simulink model "mw_autodma"  (R2020a)
settings: Solver=VariableStepAuto  StartTime=0.0  StopTime=(2*8192)/256e6  RelTol=1e-3
InitFcn:
  | fs = 256e6;
libraries: hdlsllib x5, simulink x4
settings Model: Creator=david  LastModifiedBy=david
settings OptimizationCC: BlockReduction=off  ConditionallyExecuteInputs=off  DefaultParameterBehavior=Inlined
settings DebuggingCC: AlgebraicLoopMsg=error
settings HardwareCC: ProdBitPerPointer=32  ProdBitPerSizeT=32  ProdBitPerPtrDiffT=32  ProdLargestAtomicFloat=None  ProdIntDivRoundTo=Undefined  ProdEndianess=Unspecified  ProdWordSize=32  ProdHWDeviceType=ASIC/FPGA->ASIC/FPGA  TargetBitPerPointer=64  TargetBitPerSizeT=64  TargetBitPerPtrDiffT=64  TargetLongLongMode=on  TargetIntDivRoundTo=Zero  TargetEndianess=LittleEndian  TargetWordSize=64  TargetHWDeviceType=Custom Processor->MATLAB Host Computer  ProdEqTarget=off

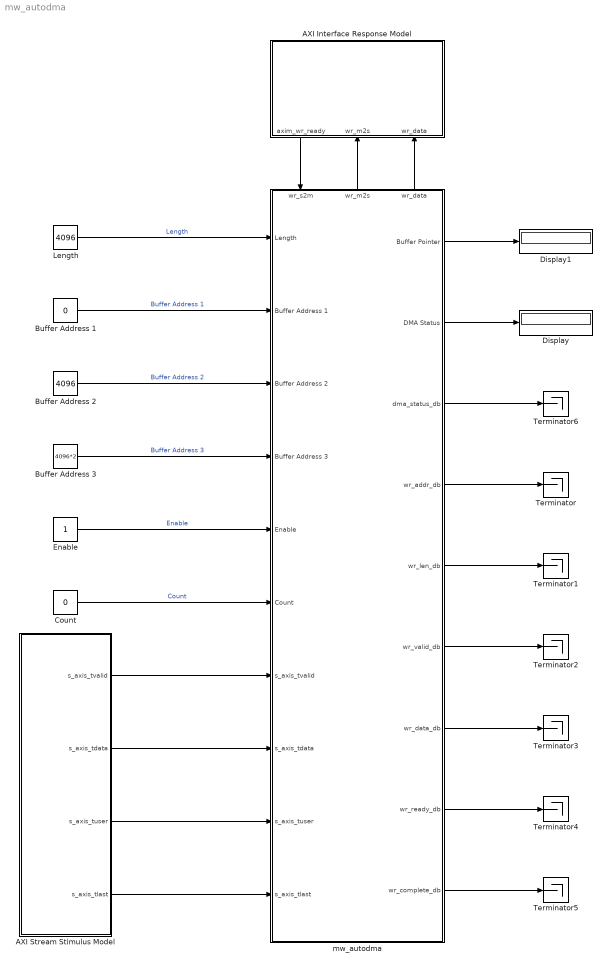
== system mw_autodma ==
  AXI Interface Response Model : Subsystem
      settings: PortSchema="{\"entries\":[{\"content\":{\"sides\":[{\"content\":{\"connectorIds\":[]},\"type\":\"ConnectorPlacement.EquallySpacedRectSide\",\"uuid\":\"6953abbe-a6d5-4686-b276-b89fe5e6bb23\"},{\"content\":{\"connectorIds\":[],\"side\":\"RIGHT\"},\"type\":\"ConnectorPlacement.EquallySpacedRectSide\",\"uuid\":\"539ff6ac-c243-4534-87d0-888ff9534a8b\"},{\"content\":{\"connectorIds\":[],\"side\":\"TOP\"},\"type\":\"ConnectorPlacement.EquallySpacedRectSide\",\"uuid\":\"8a126ba7-8eec-4733-ae4d-1ac2504ae558\"},{\"content\":{\"connectorIds\":[\"Out1\",\"In1\",\"In2\"],\"side\":\"BOTTOM\"},\"type\":\"ConnectorPlacement.EquallySpacedRectSide\",\"uuid\":\"05254abb-7168-4864-8cc1-53a55061df5a\"}]},\"type\":\"ConnectorPlacement.EquallySpacedConnector\",\"uuid\":\"821e8dd7-bdc5-437f-b697-1dcc78127ace\"}],\"packageUris\":[\"http://schema.mathworks.com/mf0/Connector/19700101\"],\"version\":\"1.0\"}"
  AXI Stream Stimulus Model : Subsystem
  Buffer Address 1 : Constant  Value=0  OutDataTypeStr=uint32  SampleTime=1/fs
  Buffer Address 2 : Constant  Value=4096  OutDataTypeStr=uint32  SampleTime=1/fs
  Buffer Address 3 : Constant  Value=4096*2  OutDataTypeStr=uint32  SampleTime=1/fs
  Count : Constant  Value=0  OutDataTypeStr=uint32  SampleTime=1/fs
  Display : Display
  Display1 : Display
  Enable : Constant  OutDataTypeStr=uint32  SampleTime=1/fs
  Length : Constant  Value=4096  OutDataTypeStr=uint32  SampleTime=1/fs
  Terminator{,1..6} (7 alike) : Terminator
  mw_autodma : Subsystem  TreatAsAtomicUnit=on
      settings: PortSchema="{\"entries\":[{\"content\":{\"sides\":[{\"content\":{\"connectorIds\":[\"In1\",\"In2\",\"In3\",\"In4\",\"In5\",\"In6\",\"In7\",\"In8\",\"In9\",\"In10\"]},\"type\":\"ConnectorPlacement.EquallySpacedRectSide\",\"uuid\":\"feed7d54-868e-4051-a23d-06bc6ab36d5c\"},{\"content\":{\"connectorIds\":[\"Out1\",\"Out2\",\"Out3\",\"Out4\",\"Out5\",\"Out6\",\"Out7\",\"Out8\",\"Out9\"],\"side\":\"RIGHT\"},\"type\":\"ConnectorPlacement.EquallySpacedRectSide\",\"uuid\":\"d3d03214-b2fe-4ae7-abfc-e707b28dda07\"},{\"content\":{\"connectorIds\":[\"In11\",\"Out10\",\"Out11\"],\"side\":\"TOP\"},\"type\":\"ConnectorPlacement.EquallySpacedRectSide\",\"uuid\":\"f475a445-5d90-4da5-970d-06e407d01a30\"}]},\"type\":\"ConnectorPlacement.EquallySpacedConnector\",\"uuid\":\"e5023fc6-91ea-4318-839d-5fb8d0ed3484\"}],\"packageUris\":[\"http://schema.mathworks.com/mf0/Connector/19700101\"],\"version\":\"1.0\"}"
  wires:
  Length/1 -> mw_autodma/1(Length)  "Length"
  Buffer Address 1/1 -> mw_autodma/2(Buffer Address 1)  "Buffer Address 1"
  Buffer Address 2/1 -> mw_autodma/3(Buffer Address 2)  "Buffer Address 2"
  Buffer Address 3/1 -> mw_autodma/4(Buffer Address 3)  "Buffer Address 3"
  Enable/1 -> mw_autodma/5(Enable)  "Enable"
  Count/1 -> mw_autodma/6(Count)  "Count"
  AXI Interface Response Model/1(axim_wr_ready) -> mw_autodma/11(wr_s2m)
  mw_autodma/11(wr_data) -> AXI Interface Response Model/2(wr_data)
  mw_autodma/4(wr_addr_db) -> Terminator/1
  mw_autodma/5(wr_len_db) -> Terminator1/1
  mw_autodma/6(wr_valid_db) -> Terminator2/1
  mw_autodma/7(wr_data_db) -> Terminator3/1
  mw_autodma/8(wr_ready_db) -> Terminator4/1
  mw_autodma/9(wr_complete_db) -> Terminator5/1
  mw_autodma/3(dma_status_db) -> Terminator6/1
  mw_autodma/2(DMA Status) -> Display/1
  mw_autodma/1(Buffer Pointer) -> Display1/1
  AXI Stream Stimulus Model/1(s_axis_tvalid) -> mw_autodma/7(s_axis_tvalid)
  AXI Stream Stimulus Model/2(s_axis_tdata) -> mw_autodma/8(s_axis_tdata)
  AXI Stream Stimulus Model/3(s_axis_tuser) -> mw_autodma/9(s_axis_tuser)
  AXI Stream Stimulus Model/4(s_axis_tlast) -> mw_autodma/10(s_axis_tlast)
  mw_autodma/10(wr_m2s) -> AXI Interface Response Model/1(wr_m2s)

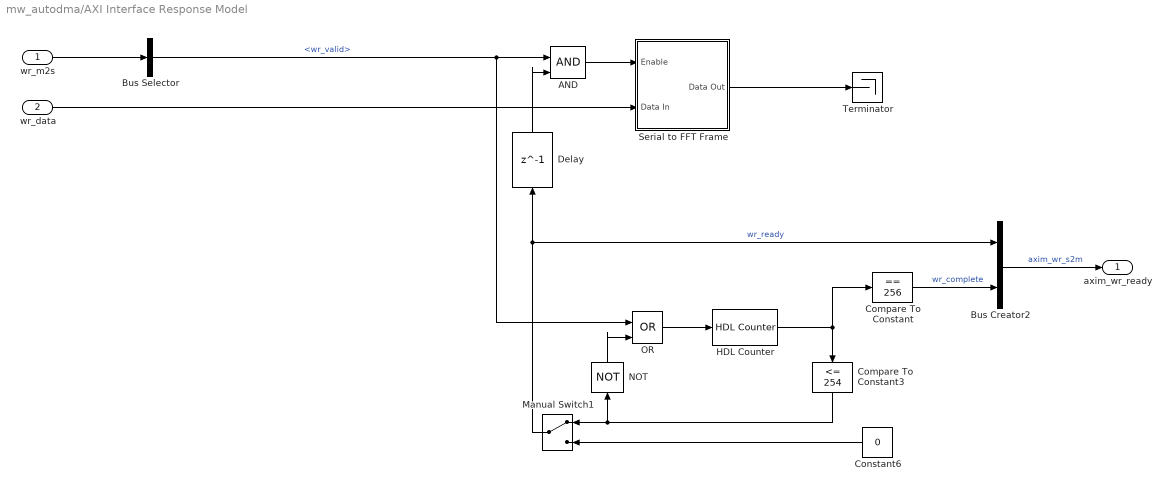
== system mw_autodma/AXI Interface Response Model ==
  wr_m2s : Inport
  wr_data : Inport  Port=2
  AND : Logic  IconShape=distinctive  AllPortsSameDT=off  OutDataTypeStr=boolean
  Bus Creator2 : BusCreator  Inputs=2
  Bus Selector : BusSelector  OutputSignals=wr_valid
  Compare To Constant : simulink/Logic and Bit Operations/Compare To Constant  relop===  const=256  OutDataTypeStr=boolean
  Compare To Constant3 : simulink/Logic and Bit Operations/Compare To Constant  relop=<=  const=254  OutDataTypeStr=boolean
  Constant6 : Constant  Value=0  OutDataTypeStr=boolean  SampleTime=-1
  Delay : Delay  DelayLength=1  InitialCondition=0  UseCircularBuffer=on
  HDL Counter : hdlsllib/Sources/HDL Counter  CountType=Count limited  CountInit=0  CountStep=1  CountMax=256  CountFromType=Initial value  CountFrom=0  CountResetPort=off  CountLoadPort=off  CountEnbPort=on  CountDirPort=off  CountDataType=Unsigned  CountWordLen=10  CountFracLen=0  CountSampTime=1
  Manual Switch1 : ManualSwitch
  NOT : Logic  Operator=NOT  IconShape=distinctive  AllPortsSameDT=off  OutDataTypeStr=boolean
  OR : Logic  Operator=OR  IconShape=distinctive  AllPortsSameDT=off  OutDataTypeStr=boolean
  Serial to FFT Frame : Subsystem  mask{N=4096}
      mask prompts: N "FFT Size:"
      mask DialogControl DescGroupVar Prompt: Serial to FFT Frame
      mask DialogControl DescTextVar Prompt: This block converts serial FFT data to a frame of FFT data. An FFT shift is applied to correct for out of order FFT data.
      mask DialogControl ParameterGroupVar Prompt: Main
  Terminator : Terminator
  axim_wr_ready : Outport
  wires:
  Delay/1 -> AND/2
  Compare To Constant/1 -> Bus Creator2/2  "wr_complete"
  Bus Selector/1 -> AND/1, OR/1  "<wr_valid>"
  AND/1 -> Serial to FFT Frame/1(Enable)
  Constant6/1 -> Manual Switch1/2
  HDL Counter/1 -> Compare To Constant3/1, Compare To Constant/1
  Compare To Constant3/1 -> NOT/1, Manual Switch1/1
  OR/1 -> HDL Counter/1
  NOT/1 -> OR/2
  Bus Creator2/1 -> axim_wr_ready/1  "axim_wr_s2m"
  Manual Switch1/1 -> Bus Creator2/1, Delay/1  "wr_ready"
  wr_m2s/1 -> Bus Selector/1
  Serial to FFT Frame/1(Data Out) -> Terminator/1
  wr_data/1 -> Serial to FFT Frame/2(Data In)

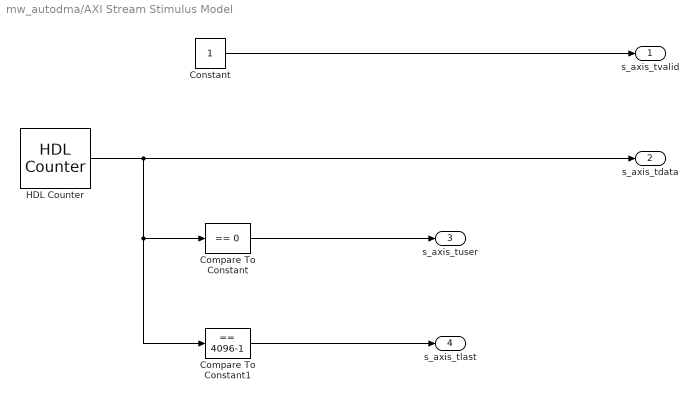
== system mw_autodma/AXI Stream Stimulus Model ==
  Compare To Constant : simulink/Logic and Bit Operations/Compare To Constant  relop===  const=0  OutDataTypeStr=boolean
  Compare To Constant1 : simulink/Logic and Bit Operations/Compare To Constant  relop===  const=4096-1  OutDataTypeStr=boolean
  Constant : Constant  OutDataTypeStr=boolean  SampleTime=-1
  HDL Counter : hdlsllib/Sources/HDL Counter  CountType=Count limited  CountInit=0  CountStep=1  CountMax=4096-1  CountFromType=Initial value  CountFrom=0  CountResetPort=off  CountLoadPort=off  CountEnbPort=off  CountDirPort=off  CountDataType=Unsigned  CountWordLen=32  CountFracLen=0  CountSampTime=-1
  s_axis_tvalid : Outport
  s_axis_tdata : Outport  Port=2
  s_axis_tuser : Outport  Port=3
  s_axis_tlast : Outport  Port=4
  wires:
  Constant/1 -> s_axis_tvalid/1
  Compare To Constant/1 -> s_axis_tuser/1
  Compare To Constant1/1 -> s_axis_tlast/1
  HDL Counter/1 -> s_axis_tdata/1, Compare To Constant1/1, Compare To Constant/1

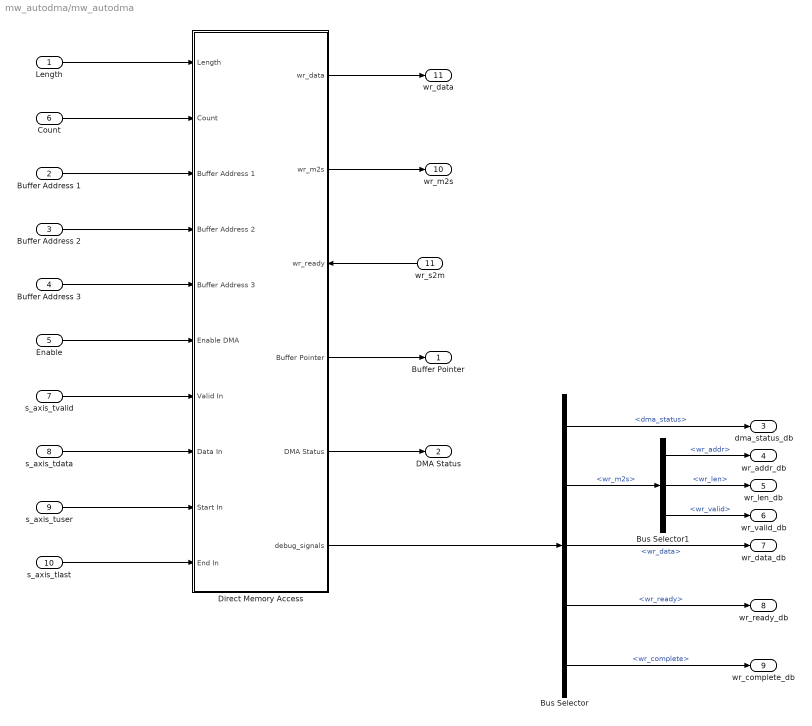
== system mw_autodma/mw_autodma ==
  Length : Inport
  Buffer Address 1 : Inport  Port=2
  Buffer Address 2 : Inport  Port=3
  Buffer Address 3 : Inport  Port=4
  Enable : Inport  Port=5
  Count : Inport  Port=6
  s_axis_tvalid : Inport  Port=7
  s_axis_tdata : Inport  Port=8
  s_axis_tuser : Inport  Port=9
  s_axis_tlast : Inport  Port=10
  wr_s2m : Inport  Port=11
  Bus Selector : BusSelector  OutputSignals=dma_status,wr_m2s,wr_data,wr_ready,wr_complete
  Bus Selector1 : BusSelector  OutputSignals=wr_addr,wr_len,wr_valid
  Direct Memory Access : Subsystem
      settings: PortSchema="{\"entries\":[{\"content\":{\"sides\":[{\"content\":{\"connectorIds\":[\"In1\",\"In2\",\"In3\",\"In4\",\"In5\",\"In6\",\"In7\",\"In8\",\"In9\",\"In10\"]},\"type\":\"ConnectorPlacement.EquallySpacedRectSide\",\"uuid\":\"00536163-74b2-48b0-a433-f45a47e82c13\"},{\"content\":{\"connectorIds\":[\"Out1\",\"Out2\",\"In11\",\"Out3\",\"Out4\",\"Out5\"],\"side\":\"RIGHT\"},\"type\":\"ConnectorPlacement.EquallySpacedRectSide\",\"uuid\":\"bb0450ed-1752-4cb2-9c7c-352c8b1a90c1\"},{\"content\":{\"connectorIds\":[],\"side\":\"TOP\"},\"type\":\"ConnectorPlacement.EquallySpacedRectSide\",\"uuid\":\"451bf01f-2efb-42e7-aace-9484eb9026e5\"}]},\"type\":\"ConnectorPlacement.EquallySpacedConnector\",\"uuid\":\"5c52148d-823b-46a6-a578-8e88341097d4\"}],\"packageUris\":[\"http://schema.mathworks.com/mf0/Connector/19700101\"],\"version\":\"1.0\"}"
  Buffer Pointer : Outport
  DMA Status : Outport  Port=2
  dma_status_db : Outport  Port=3
  wr_addr_db : Outport  Port=4
  wr_len_db : Outport  Port=5
  wr_valid_db : Outport  Port=6
  wr_data_db : Outport  Port=7
  wr_ready_db : Outport  Port=8
  wr_complete_db : Outport  Port=9
  wr_m2s : Outport  Port=10
  wr_data : Outport  Port=11
  wires:
  Direct Memory Access/4(DMA Status) -> DMA Status/1
  Count/1 -> Direct Memory Access/2(Count)
  s_axis_tlast/1 -> Direct Memory Access/10(End In)
  Bus Selector1/3 -> wr_valid_db/1  "<wr_valid>"
  s_axis_tvalid/1 -> Direct Memory Access/7(Valid In)
  s_axis_tdata/1 -> Direct Memory Access/8(Data In)
  s_axis_tuser/1 -> Direct Memory Access/9(Start In)
  Bus Selector/5 -> wr_complete_db/1  "<wr_complete>"
  Direct Memory Access/2(wr_m2s) -> wr_m2s/1
  Bus Selector1/1 -> wr_addr_db/1  "<wr_addr>"
  Bus Selector1/2 -> wr_len_db/1  "<wr_len>"
  Bus Selector/4 -> wr_ready_db/1  "<wr_ready>"
  Bus Selector/2 -> Bus Selector1/1  "<wr_m2s>"
  Bus Selector/3 -> wr_data_db/1  "<wr_data>"
  Buffer Address 1/1 -> Direct Memory Access/3(Buffer Address 1)
  Bus Selector/1 -> dma_status_db/1  "<dma_status>"
  Enable/1 -> Direct Memory Access/6(Enable DMA)
  Direct Memory Access/5(debug_signals) -> Bus Selector/1
  Direct Memory Access/1(wr_data) -> wr_data/1
  Direct Memory Access/3(Buffer Pointer) -> Buffer Pointer/1
  wr_s2m/1 -> Direct Memory Access/11(wr_ready)
  Length/1 -> Direct Memory Access/1(Length)
  Buffer Address 2/1 -> Direct Memory Access/4(Buffer Address 2)
  Buffer Address 3/1 -> Direct Memory Access/5(Buffer Address 3)

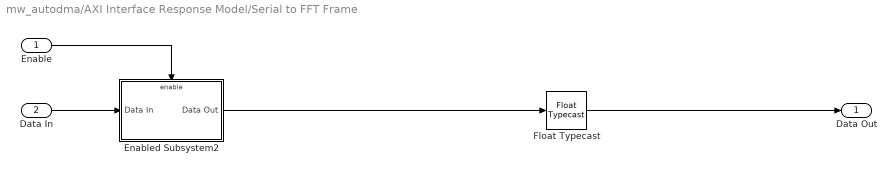
== system mw_autodma/AXI Interface Response Model/Serial to FFT Frame ==
  Enable : Inport
  Data In : Inport  Port=2
  Enabled Subsystem2 : Subsystem  TreatAsAtomicUnit=on
  Float Typecast : FloatTypecast
  Data Out : Outport
  wires:
  Float Typecast/1 -> Data Out/1
  Data In/1 -> Enabled Subsystem2/1(Data In)
  Enable/1 -> Enabled Subsystem2/Enable
  Enabled Subsystem2/1(Data Out) -> Float Typecast/1

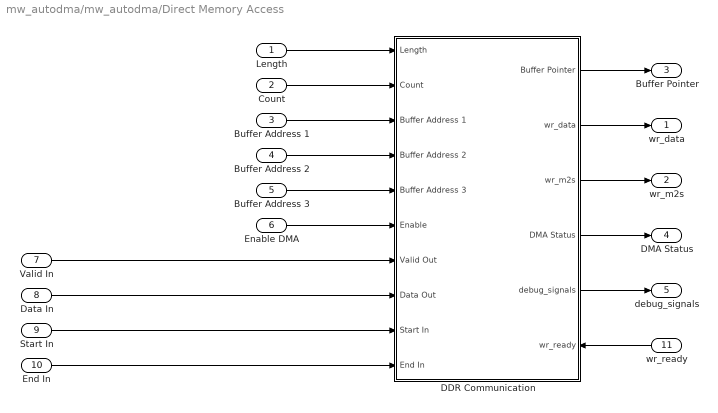
== system mw_autodma/mw_autodma/Direct Memory Access ==
  Length : Inport
  Count : Inport  Port=2
  Buffer Address 1 : Inport  Port=3
  Buffer Address 2 : Inport  Port=4
  Buffer Address 3 : Inport  Port=5
  Enable DMA : Inport  Port=6
  Valid In : Inport  Port=7
  Data In : Inport  Port=8
  Start In : Inport  Port=9
  End In : Inport  Port=10
  wr_ready : Inport  Port=11
  DDR Communication : Subsystem
      settings: PortSchema="{\"entries\":[{\"content\":{\"sides\":[{\"content\":{\"connectorIds\":[\"In1\",\"In2\",\"In3\",\"In4\",\"In5\",\"In6\",\"In7\",\"In8\",\"In9\",\"In10\"]},\"type\":\"ConnectorPlacement.EquallySpacedRectSide\",\"uuid\":\"1b0605ed-f994-4b4f-952c-c7a4534a55db\"},{\"content\":{\"connectorIds\":[\"Out1\",\"Out2\",\"Out3\",\"Out4\",\"Out5\",\"In11\"],\"side\":\"RIGHT\"},\"type\":\"ConnectorPlacement.EquallySpacedRectSide\",\"uuid\":\"e00ce3f0-150b-4c4f-a18d-f280380b0728\"},{\"content\":{\"connectorIds\":[],\"side\":\"TOP\"},\"type\":\"ConnectorPlacement.EquallySpacedRectSide\",\"uuid\":\"b0ef8b1e-3f6b-405f-8824-c1fb25b076ef\"}]},\"type\":\"ConnectorPlacement.EquallySpacedConnector\",\"uuid\":\"53c75551-9c59-440c-835f-2065b8683bc1\"}],\"packageUris\":[\"http://schema.mathworks.com/mf0/Connector/19700101\"],\"version\":\"1.0\"}"
  wr_data : Outport
  wr_m2s : Outport  Port=2
  Buffer Pointer : Outport  Port=3
  DMA Status : Outport  Port=4
  debug_signals : Outport  Port=5
  wires:
  Count/1 -> DDR Communication/2(Count)
  DDR Communication/5(debug_signals) -> debug_signals/1
  Length/1 -> DDR Communication/1(Length)
  DDR Communication/4(DMA Status) -> DMA Status/1
  Enable DMA/1 -> DDR Communication/6(Enable)
  Buffer Address 3/1 -> DDR Communication/5(Buffer Address 3)
  Buffer Address 2/1 -> DDR Communication/4(Buffer Address 2)
  Buffer Address 1/1 -> DDR Communication/3(Buffer Address 1)
  Valid In/1 -> DDR Communication/7(Valid Out)
  DDR Communication/1(Buffer Pointer) -> Buffer Pointer/1
  Data In/1 -> DDR Communication/8(Data Out)
  End In/1 -> DDR Communication/10(End In)
  Start In/1 -> DDR Communication/9(Start In)
  DDR Communication/3(wr_m2s) -> wr_m2s/1
  DDR Communication/2(wr_data) -> wr_data/1
  wr_ready/1 -> DDR Communication/11(wr_ready)

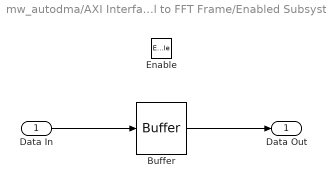
== system mw_autodma/AXI Interface Response Model/Serial to FFT Frame/Enabled Subsystem2 ==
  Data In : Inport
  Enable : EnablePort
  Buffer : Buffer  N=N  OutputFrames=off
  Data Out : Outport
  wires:
  Buffer/1 -> Data Out/1
  Data In/1 -> Buffer/1

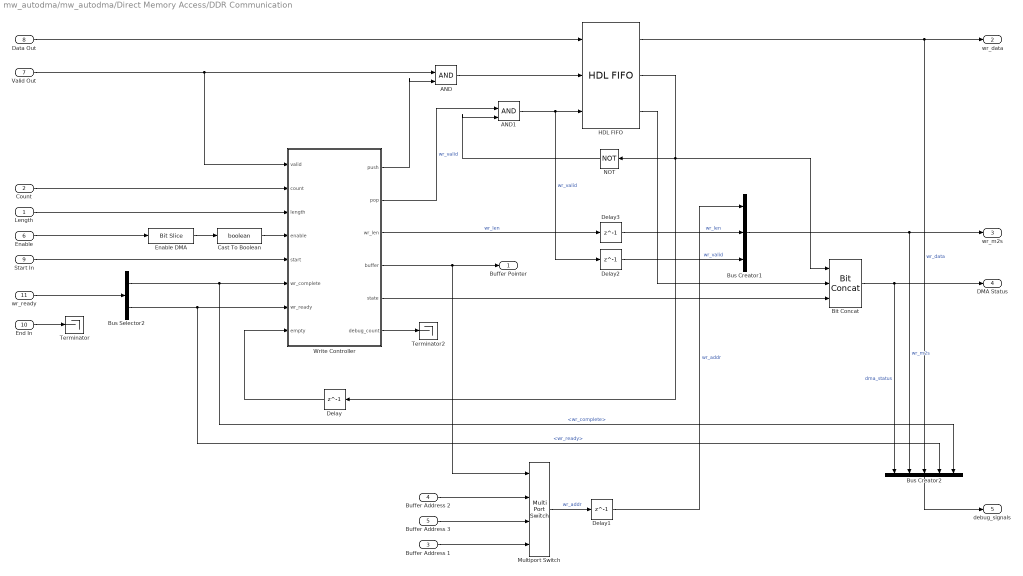
== system mw_autodma/mw_autodma/Direct Memory Access/DDR Communication ==
  Length : Inport
  Count : Inport  Port=2
  Buffer Address 1 : Inport  Port=3
  Buffer Address 2 : Inport  Port=4
  Buffer Address 3 : Inport  Port=5
  Enable : Inport  Port=6
  Valid Out : Inport  Port=7
  Data Out : Inport  Port=8
  Start In : Inport  Port=9
  End In : Inport  Port=10
  wr_ready : Inport  Port=11
  AND : Logic  IconShape=distinctive  AllPortsSameDT=off  OutDataTypeStr=boolean
  AND1 : Logic  IconShape=distinctive  AllPortsSameDT=off  OutDataTypeStr=boolean
  Bit Concat : hdlsllib/Logic and Bit Operations/Bit Concat  numInputs=3
  Bus Creator1 : BusCreator  Inputs=3
  Bus Creator2 : BusCreator  Inputs=5
  Bus Selector2 : BusSelector  OutputSignals=wr_complete,wr_ready
  Cast To Boolean : DataTypeConversion  OutDataTypeStr=boolean
  Delay{,1..3} (4 alike) : Delay  DelayLength=1
  Enable DMA : hdlsllib/Logic and Bit Operations/Bit Slice  lidx=0  ridx=0
      settings: SourceProductBaseCode=SL
  HDL FIFO : hdlsllib/HDL RAMs/HDL FIFO  fifo_size=4096  mode=Classic  ratio=1  push_msg=Error  pop_msg=Error  show_empty=on  show_full=on  show_num=off  LabelModeActiveChoice_Mode=Classic
      settings: SourceProductBaseCode=SL
  Multiport Switch : MultiPortSwitch  DataPortOrder=Zero-based contiguous  zeroidx=on
  NOT : Logic  Operator=NOT  IconShape=distinctive  AllPortsSameDT=off  OutDataTypeStr=boolean
  Terminator : Terminator
  Terminator2 : Terminator
  Write Controller : MATLAB Function  TreatAsAtomicUnit=on
  Buffer Pointer : Outport
  wr_data : Outport  Port=2
  wr_m2s : Outport  Port=3  VectorParamsAs1DForOutWhenUnconnected=off
  DMA Status : Outport  Port=4
  debug_signals : Outport  Port=5
  wires:
  Delay3/1 -> Bus Creator1/2  "wr_len"
  Delay2/1 -> Bus Creator1/3  "wr_valid"
  Delay1/1 -> Bus Creator1/1  "wr_addr"
  Write Controller/3(wr_len) -> Delay3/1  "wr_len"
  Bus Selector2/1 -> Write Controller/6(wr_complete), Bus Creator2/5  "<wr_complete>"
  Count/1 -> Write Controller/2(count)
  Bus Creator2/1 -> debug_signals/1
  Cast To Boolean/1 -> Write Controller/4(enable)
  Enable DMA/1 -> Cast To Boolean/1
  Bus Selector2/2 -> Bus Creator2/4, Write Controller/7(wr_ready)  "<wr_ready>"
  Write Controller/2(pop) -> AND1/1  "wr_valid"
  Start In/1 -> Write Controller/5(start)
  Write Controller/6(debug_count) -> Terminator2/1
  Length/1 -> Write Controller/3(length)
  HDL FIFO/3 -> Bit Concat/2
  Write Controller/5(state) -> Bit Concat/3
  Bit Concat/1 -> DMA Status/1, Bus Creator2/1  "dma_status"
  Write Controller/4(buffer) -> Multiport Switch/1, Buffer Pointer/1
  End In/1 -> Terminator/1
  Enable/1 -> Enable DMA/1
  HDL FIFO/2 -> NOT/1, Bit Concat/1, Delay/1
  AND/1 -> HDL FIFO/2
  Valid Out/1 -> AND/1, Write Controller/1(valid)
  HDL FIFO/1 -> wr_data/1, Bus Creator2/3  "wr_data"
  Write Controller/1(push) -> AND/2
  Bus Creator1/1 -> wr_m2s/1, Bus Creator2/2  "wr_m2s"
  wr_ready/1 -> Bus Selector2/1
  AND1/1 -> HDL FIFO/3, Delay2/1  "wr_valid"
  NOT/1 -> AND1/2
  Data Out/1 -> HDL FIFO/1
  Delay/1 -> Write Controller/8(empty)
  Multiport Switch/1 -> Delay1/1  "wr_addr"
  Buffer Address 1/1 -> Multiport Switch/4
  Buffer Address 2/1 -> Multiport Switch/2
  Buffer Address 3/1 -> Multiport Switch/3

== matlab function mw_autodma/Direct Memory Access/DDR Communication/Write Controller ==
  data: valid input; count input; push output boolean; pop output; length input; enable input; start input boolean; wr_complete input; wr_ready input; wr_len output; buffer output; state output; empty input; debug_count output
function [push, pop, wr_len, buffer, state, debug_count] = ddr_write_control(valid, count, length, enable, start, wr_complete, wr_ready, empty)

% Create persistent variables (registers)
persistent burst_count;
persistent time_count;
persistent current_state;
persistent buffer_pointer;

if(isempty(burst_count))
    burst_count = fi(0, 0, 16, 0);
end

if(isempty(time_count))
    time_count = fi(0, 0, 32, 0);
end

if(isempty(current_state))
    current_state = fi(0, 0, 4, 0);
end

if(isempty(buffer_pointer))
    buffer_pointer = fi(0, 0, 2, 0);
end

% FSM States
IDLE  = fi(0, 0, 4, 0);
START = fi(1, 0, 4, 0);
COUNT = fi(2, 0, 4, 0);
WAIT  = fi(4, 0, 4, 0);

switch current_state
    case IDLE
        push = false;
        pop = wr_ready;
        wr_len = length;
        buffer = buffer_pointer;
        state = current_state;
        debug_count = burst_count;
        
        burst_count = fi(0, 0, 16, 0);
        
        if enable && time_count >= count
            current_state = START;
            time_count = fi(0, 0, 32, 0);
        else
            current_state = IDLE;
            if time_count < count
                time_count = fi(time_count + 1, 0, 32, 0);
            end
        end
        
    case START
        pop = false;
        wr_len = length;
        buffer = buffer_pointer;
        state = current_state;
        debug_count = burst_count;
        
        if ~enable
            push = false;
            burst_count = fi(0, 0, 16, 0);
            current_state = IDLE;
        else
            if start && valid
                push = true;
                burst_count = fi(burst_count + 1, 0, 16, 0);
                current_state = COUNT;
            else
                push = false;
                burst_count = fi(0, 0, 16, 0);
                current_state = START;
            end
        end            
        
    case COUNT
        pop = false;
        wr_len = length;
        buffer = buffer_pointer;
        state = current_state;
        debug_count = burst_count;
        
        if valid
            push = true;
            burst_count = fi(burst_count + 1, 0, 16, 0);
        else
            push = false;
        end
        
        if burst_count >= length
            current_state = WAIT;
            if buffer_pointer > fi(1, 0, 2, 0)
                buffer_pointer = fi(0, 0, 2, 0);
            else
            	buffer_pointer = fi(buffer_pointer+1, 0, 2, 0);
            end
        else
            current_state = COUNT;
        end
        
    case WAIT
        push = false;
        pop = wr_ready;
        wr_len = length;
        buffer = buffer_pointer;
        state = current_state;
        debug_count = burst_count;
        
        burst_count = fi(0, 0, 16, 0);
        
        if empty && wr_complete
            current_state = IDLE;
        else
            current_state = WAIT;
        end
        
    otherwise
        push = false;
        pop = wr_ready;
        wr_len = length;
        buffer = buffer_pointer;
        state = current_state;
        debug_count = burst_count;
        
        burst_count = fi(0, 0, 16, 0);
        
        current_state = IDLE;
        
end
